simulink model "sch_pendule_etudiant_2016_LQR"  (R2016a)
settings: Solver=VariableStepAuto  StartTime=0.0  StopTime=10.0  RelTol=1e-3
values from neighbouring files (symbols this model uses):
  CH = struct()    [prg_pendule_etudiant.m]
settings Model: Creator=ygorra  LastModifiedBy=hp
settings ConfigComp: CovModelRefEnable=Off

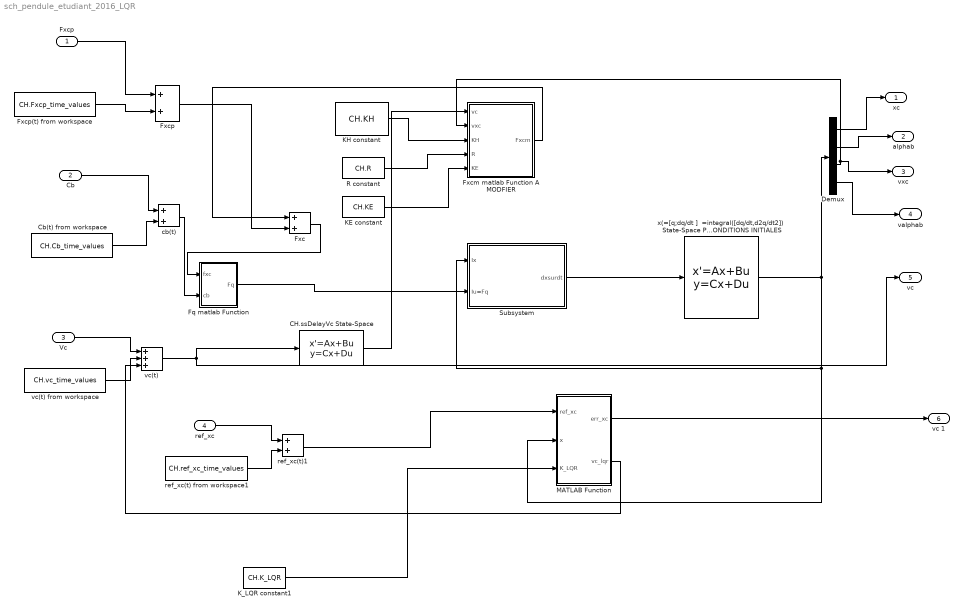
== system sch_pendule_etudiant_2016_LQR ==
  "Fxcp " : Inport
  "Cb " : Inport  Port=2
  "Vc  " : Inport  Port=3
  "ref_xc  " : Inport  Port=4
  " Fq matlab Function" : MATLAB Function  TreatAsAtomicUnit=on
  CH.ssDelayVc State-Space : StateSpace  A=CH.ssDelayVc.A  B=CH.ssDelayVc.B  C=CH.ssDelayVc.C  D=CH.ssDelayVc.D  X0=0
  Cb(t) from workspace : FromWorkspace  VariableName=CH.Cb_time_values  SampleTime=0  OutputAfterFinalValue=Holding final value
  Demux : Demux
  Fxc : Sum
  Fxcm matlab Function A MODFIER : MATLAB Function  TreatAsAtomicUnit=on
  Fxcp : Sum
  Fxcp(t) from workspace : FromWorkspace  VariableName=CH.Fxcp_time_values  SampleTime=0  OutputAfterFinalValue=Holding final value
  KE constant : Constant  Value=CH.KE
  KH constant : Constant  Value=CH.KH
  K_LQR constant1 : Constant  Value=CH.K_LQR  VectorParams1D=off
  MATLAB Function : MATLAB Function  TreatAsAtomicUnit=on
  R constant : Constant  Value=CH.R
  Subsystem : Subsystem
  cb(t) : Sum
  ref_xc(t) from workspace1 : FromWorkspace  VariableName=CH.ref_xc_time_values  SampleTime=0  OutputAfterFinalValue=Holding final value
  ref_xc(t)1 : Sum
  vc(t) : Sum  Inputs=+++
  vc(t) from workspace : FromWorkspace  VariableName=CH.vc_time_values  SampleTime=0  OutputAfterFinalValue=Holding final value
  x(=[q;dq/dt ]  =integral([dq/dt,d2q/dt2]) State-Space PROGRAMMER INTEGRATEUR A 4 ENTREES ET AJOUTER CONDITIONS INITIALES : StateSpace  A=zeros(4,4)  B=eye(4,4)  C=eye(4,4)  D=zeros(4,4)  X0=[CH.xc_init;CH.alphab_init;CH.vxc_init;CH.valphab_init]
  xc : Outport
  alphab : Outport  Port=2
  vxc : Outport  Port=3
  valphab : Outport  Port=4
  "vc " : Outport  Port=5
  vc 1 : Outport  Port=6
  wires:
  KH constant/1 -> Fxcm matlab Function A MODFIER/3(KH)
  R constant/1 -> Fxcm matlab Function A MODFIER/4(R)
  KE constant/1 -> Fxcm matlab Function A MODFIER/5(KE)
  Fxcm matlab Function A MODFIER/1(Fxcm) -> Fxc/1
  Fxcp/1 -> Fxc/2
  Fxc/1 -> " Fq matlab Function"/1(fxc)
  vc(t) from workspace/1 -> vc(t)/2
  "Vc  "/1 -> vc(t)/1
  x(=[q;dq/dt ]  =integral([dq/dt,d2q/dt2]) State-Space PROGRAMMER INTEGRATEUR A 4 ENTREES ET AJOUTER CONDITIONS INITIALES/1 -> MATLAB Function/2(x), Subsystem/1(Ix), Demux/1
  "Fxcp "/1 -> Fxcp/1
  "Cb "/1 -> cb(t)/1
  Fxcp(t) from workspace/1 -> Fxcp/2
  Cb(t) from workspace/1 -> cb(t)/2
  cb(t)/1 -> " Fq matlab Function"/2(cb)
  Demux/1 -> xc/1
  Demux/2 -> alphab/1
  vc(t)/1 -> "vc "/1, CH.ssDelayVc State-Space/1
  CH.ssDelayVc State-Space/1 -> Fxcm matlab Function A MODFIER/1(vc)
  Demux/3 -> Fxcm matlab Function A MODFIER/2(vxc), vxc/1
  Demux/4 -> valphab/1
  " Fq matlab Function"/1(Fq) -> Subsystem/2(Iu=Fq)
  Subsystem/1(dxsurdt) -> x(=[q;dq/dt ]  =integral([dq/dt,d2q/dt2]) State-Space PROGRAMMER INTEGRATEUR A 4 ENTREES ET AJOUTER CONDITIONS INITIALES/1
  ref_xc(t) from workspace1/1 -> ref_xc(t)1/2
  "ref_xc  "/1 -> ref_xc(t)1/1
  MATLAB Function/2(vc_lqr) -> vc(t)/3
  ref_xc(t)1/1 -> MATLAB Function/1(ref_xc)
  K_LQR constant1/1 -> MATLAB Function/3(K_LQR)
  MATLAB Function/1(err_xc) -> vc 1/1

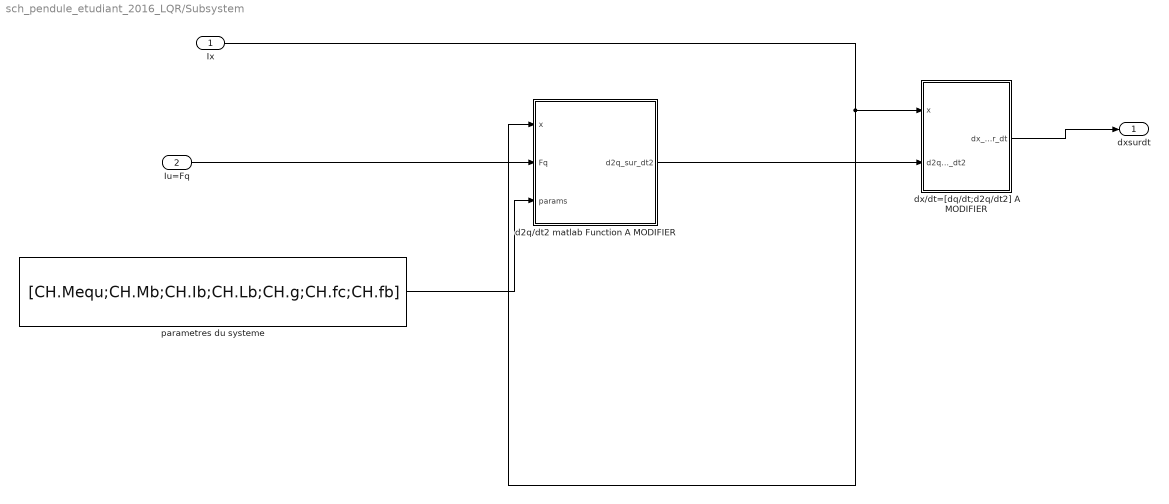
== system sch_pendule_etudiant_2016_LQR/Subsystem ==
  Ix : Inport
  Iu=Fq : Inport  Port=2
  " dx/dt=[dq/dt;d2q/dt2] A MODIFIER " : MATLAB Function  TreatAsAtomicUnit=on
  d2q/dt2 matlab Function A MODIFIER : MATLAB Function  TreatAsAtomicUnit=on
  parametres du systeme : Constant  Value=[CH.Mequ;CH.Mb;CH.Ib;CH.Lb;CH.g;CH.fc;CH.fb]
  dxsurdt : Outport
  wires:
  parametres du systeme/1 -> d2q/dt2 matlab Function A MODIFIER/3(params)
  " dx/dt=[dq/dt;d2q/dt2] A MODIFIER "/1(dx_sur_dt) -> dxsurdt/1
  d2q/dt2 matlab Function A MODIFIER/1(d2q_sur_dt2) -> " dx/dt=[dq/dt;d2q/dt2] A MODIFIER "/2(d2q_sur_dt2)
  Iu=Fq/1 -> d2q/dt2 matlab Function A MODIFIER/2(Fq)
  Ix/1 -> d2q/dt2 matlab Function A MODIFIER/1(x), " dx/dt=[dq/dt;d2q/dt2] A MODIFIER "/1(x)

== matlab function sch_pendule_etudiant_2016_LQR/Fxcm matlab Function A MODFIER ==
  data: vc input; vxc input; KH input; R input; KE input; Fxcm output
function Fxcm =clc_moteur(vc,vxc,KH,R,KE)
%calcul de Fxcm = fct(vc =tension commande, vxc =dxc/dt, parametres ) 
  Um=KH*vc; % tension d'induit moteur en V
  E=KE*vxc;% f.c.e.m en V
  I=(Um-E)/R;% courant induit en A
  Fxcm=KE*I; % Force sur le chariot en N
 
end

== matlab function sch_pendule_etudiant_2016_LQR/Subsystem/d2q//dt2 matlab Function A MODIFIER ==
  data: x input; Fq input; d2q_sur_dt2 output; params input
function d2q_sur_dt2=clc_accq(x,Fq,params)
%calcul de d2q_sur_dt2 =d2q/dt2 = fct(x, Fq , params=[Mequ,Mb,Ib,Lb,g,fc,fb] )
% principe : calculer A et H
% en deduire d2q_sur_dt2 par inversion de matrice
% 1- extraction de xc, alphab, vxc=dxc/dt, valphab
  xc=x(1);    % A MODIFIER
  alphab=x(2);% A MODIFIER
  vxc=x(3);% A MODIFIER
  valphab=x(4);% A MODIFIER
% 2- extraction des parametres
%[CH.Mequ;CH.Mb;CH.Ib;CH.Lb;CH.g;CH.fc;CH.fb]
  Mequ=params(1);
  Mb=params(2);
  Ib=params(3);
  Lb=params(4);
  g=params(5);
  fc=params(6);
  fb=params(7);
% 3-calcul des composantes de la matrice A :2X2
  A11=Mequ+Mb;
  A12=-Lb*Mb*sin(alphab);
  A21=A12;
  A22=Ib;
  A=[A11,A12;A21,A22];
% 4-calcul des composantes de H :2X1
  H1=fc*vxc;
  H2=fb*valphab+Mb*Lb*g*cos(alphab);
  H=[H1;H2];
  % A MODIFIER : determination de A,H, puis d2q_sur_dt2
  d2q_sur_dt2=pinv(A)*(Fq-H);
end

== matlab function sch_pendule_etudiant_2016_LQR/ Fq matlab Function ==
  data: fxc input; Fq output; cb input
function Fq=Fq_(fxc,cb)
  Fq=[fxc;cb];
end

== matlab function sch_pendule_etudiant_2016_LQR/Subsystem/ dx//dt=[dq//dt;d2q//dt2] A MODIFIER  ==
  data: x input; dx_sur_dt output; d2q_sur_dt2 input
function dx_sur_dt=clc_dx_sur_dt(x,d2q_sur_dt2)
  dq_sur_dt=x(3:4,1);
  dx_sur_dt=[dq_sur_dt;d2q_sur_dt2];
end

== matlab function sch_pendule_etudiant_2016_LQR/MATLAB Function ==
  data: err_xc output; ref_xc input; vc_lqr output; x input; K_LQR input
function [err_xc,vc_lqr]=vc_lqr(ref_xc,x, K_LQR)
%#codegen
x_ref=[ref_xc;pi/2;0;0];
xc=x(1);
delta_x=x_ref-x;
err_xc=ref_xc-xc;
vc_lqr=K_LQR*delta_x;
